simulink model "TBRe18_ECU_V6"  (R2015b)
settings: Solver=FixedStepDiscrete  SolverMode=SingleTasking  StartTime=0.0  StopTime=inf  FixedStep=0.0001  RelTol=1e-3
PostLoadFcn:
  | model_init();
libraries: simulink x20, simulink_extras x1
(part 3 of 4)

== system TBRe18_ECU_V6/Low_Priority_CAN_TX/ECU_Data ==
  In1 : Inport
  Bus Selector : BusSelector  OutputSignals=Input_Data_Bus.BMS_Data.Pre_Charge_Hold,Vehicle_Operation_Data.Throttle_Bool,Vehicle_Operation_Data.MCU_NMT_Mode,Vehicle_Operation_Data.PWM,Vehicle_Operation_Data.Buzzer,Vehicle_Operation_Data.Operation_Mode,Vehicle_Operation_Data.Brake_Bool
  Bus Selector1 : BusSelector  OutputSignals=Input_Data_Bus.ECU_IO_Data.Pedal_Box_Data.Brake_Voltage,Input_Data_Bus.ECU_IO_Data.Pedal_Box_Data.Throttle2_Voltage,Input_Data_Bus.ECU_IO_Data.Pedal_Box_Data.Throttle1_Voltage,Input_Data_Bus.ECU_IO_Data.Pedal_Box_Data.Throttle_%,Input_Data_Bus.ECU_IO_Data.Pedal_Box_Data.APPS_Implausibility,Input_Data_Bus.ECU_IO_Data.Pedal_Box_Data.APPS_BP_Implausibility,Input_Data_Bus.ECU_IO_Data.Pedal_Box_Data.Brake_%,Input_Data_Bus.ECU_IO_Data.Pedal_Box_Data.Throttle2_%,Input_Data_Bus.ECU_IO_Data.Pedal_Box_Data.Throttle1_%,Input_Data_Bus.ECU_IO_Data.Pedal_Box_Data.Pedal_Sensor_Fail,Input_Data_Bus.ECU_IO_Data.LV_Battery_Data.LV_Battery_Warning,Input_Data_Bus.ECU_IO_Data.LV_Battery_Data.LV_Battery_SOC,Input_Data_Bus.ECU_IO_Data.LV_Battery_Data.LV_Battery_Voltage,Input_Data_Bus.Raw_Input_Data.Hardwired_Inputs.Console_Data.Push_to_Start,Input_Data_Bus.Raw_Input_Data.Hardwired_Inputs.Console_Data.Reset
  Bus Selector2 : BusSelector  OutputSignals=Input_Data_Bus.BMS_Data.IMD_Fault,Input_Data_Bus.MCU_Data.MCU_Error,Input_Data_Bus.Raw_Input_Data.LP_CAN_RX.Shutdown_Data.BMS_Fault,Input_Data_Bus.ECU_IO_Data.Pedal_Box_Data.APPS_Implausibility,Input_Data_Bus.ECU_IO_Data.Pedal_Box_Data.APPS_BP_Implausibility,Input_Data_Bus.Shutdown_Data.Shutdown_Error,Input_Data_Bus.ECU_IO_Data.LV_Battery_Data.LV_Battery_Warning
  CanTx : S-Function  FunctionName=NsiCan_Tx  Parameters=data_can,channel,msg_name,ident,ident_type,dlc,signals  SFunctionDeploymentMode=off  EnableBusSupport=off  mask(MUXlink Can Tx){data_can=1;HIGH_SPEED;500Kbps;120 Ohm;C:\Users\William\Documents\ECU\DBC\TBRe18_DBC_V1.dbc;0;1;HIGH_SPEED;500Kbps;120 Ohm;C:\Users\William\Documents\ECU\DBC\TBRe18_DBC_V1.dbc;0;0;HIGH_SPEED;500Kbps;120 Ohm;C:\Users\l\Desktop\FYP\ECU\DBC\TBRe_DBC_V2.dbc;0;0;HIGH_SPEED;500Kbps;120 Ohm;D:\TOOLS\MUXLINK\R2011b\MUXlink\misc\j1939_adapt.dbc;0;0;HIGH_SPEED;1000Kbps;No;D:\TOOLS\MUXLINK\R2011b\MUXlink\misc\BASE_CAN_MUXLAB4.dbc;0, channel=2, msg_name=ECU_Pedal_Box_Data, ident=0x702, ident_type=STD, dlc=5, signals=Throttle_Percentage;1;32;8;APPS_Implausibility;1;4;1;APPS_BP_Implausibility;1;3;1;Brake_Percentage;1;24;8;Throttle2_Percentage;1;16;8;Throttle1_Percent;1;8;8;Pedal_Sensor_Fail;1;0;3}
      mask prompts: data_can "data can"; msg_name "msg name"
      mask help: Transmit a frame on a CAN Channel.
      mask init:
      | NsiCan_Tx_InitializationFcn();
      settings: OpenFcn=NsiCan_Tx_OpenFcn();
      mask Help:
      | eval('block=get_param(gcb, ''RTWdata'');')
      | web([docroot '\toolbox\MUXlink\html\blocks/' block.MUXlink_BlockType '.html'])
      mask Callback data_can: NsiCan_Tx_ApplyFcn(1);
      mask Callback channel: NsiCan_Tx_ApplyFcn(2);
      mask Callback msg_name: NsiCan_Tx_ApplyFcn(3);
      mask Callback ident: NsiCan_Tx_ApplyFcn(4);
      mask Callback ident_type: NsiCan_Tx_ApplyFcn(5);
      mask Callback dlc: NsiCan_Tx_ApplyFcn(6);
      mask Callback signals: NsiCan_Tx_ApplyFcn(7);
      mask Display: image(imread('nsi.bmp'));text(0.5, 0.1, 'TX_ECU_Pedal_Box_Data_CAN2', 'horizontalAlignment', 'center', 'verticalAlignment', 'base');plot([0.05 0.05 0.05 0.05 0.05 0.05 0.05 0.05 0.05 0.05]); port_label('input',1, 'Throttle_Percentage'); port_label('input',2, 'APPS_Implausibility'); port_label('input',3, 'APPS_BP_Implausibility'); port_label('input',4, 'Brake_Percentage'); port_label('input',5, 'Throttle2_Percentage'); port_label('input',6, 'Throttle1_Percent'); port_label('input',7, 'Pedal_Sensor_Fail');
  CanTx1 : S-Function  FunctionName=NsiCan_Tx  Parameters=data_can,channel,msg_name,ident,ident_type,dlc,signals  SFunctionDeploymentMode=off  EnableBusSupport=off  mask(MUXlink Can Tx){data_can=1;HIGH_SPEED;500Kbps;120 Ohm;C:\Users\William\Documents\ECU\DBC\TBRe18_DBC_V1.dbc;0;1;HIGH_SPEED;500Kbps;120 Ohm;C:\Users\William\Documents\ECU\DBC\TBRe18_DBC_V1.dbc;0;0;HIGH_SPEED;500Kbps;120 Ohm;C:\Users\l\Desktop\FYP\ECU\DBC\TBRe_DBC_V2.dbc;0;0;HIGH_SPEED;500Kbps;120 Ohm;D:\TOOLS\MUXLINK\R2011b\MUXlink\misc\j1939_adapt.dbc;0;0;HIGH_SPEED;1000Kbps;No;D:\TOOLS\MUXLINK\R2011b\MUXlink\misc\BASE_CAN_MUXLAB4.dbc;0, channel=2, msg_name=ECU_Pedal_Voltages, ident=0x703, ident_type=STD, dlc=8, signals=Brake_Voltage;1;32;16;Throttle2_Voltage;1;48;16;Throttle1_Voltage;1;0;16}
      mask prompts: data_can "data can"; msg_name "msg name"
      mask help: Transmit a frame on a CAN Channel.
      mask init:
      | NsiCan_Tx_InitializationFcn();
      settings: OpenFcn=NsiCan_Tx_OpenFcn();
      mask Help:
      | eval('block=get_param(gcb, ''RTWdata'');')
      | web([docroot '\toolbox\MUXlink\html\blocks/' block.MUXlink_BlockType '.html'])
      mask Callback data_can: NsiCan_Tx_ApplyFcn(1);
      mask Callback channel: NsiCan_Tx_ApplyFcn(2);
      mask Callback msg_name: NsiCan_Tx_ApplyFcn(3);
      mask Callback ident: NsiCan_Tx_ApplyFcn(4);
      mask Callback ident_type: NsiCan_Tx_ApplyFcn(5);
      mask Callback dlc: NsiCan_Tx_ApplyFcn(6);
      mask Callback signals: NsiCan_Tx_ApplyFcn(7);
      mask Display: image(imread('nsi.bmp'));text(0.5, 0.1, 'TX_ECU_Pedal_Voltages_CAN2', 'horizontalAlignment', 'center', 'verticalAlignment', 'base');plot([0.05 0.05 0.05 0.05 0.05 0.05 0.05 0.05 0.05 0.05]); port_label('input',1, 'Brake_Voltage'); port_label('input',2, 'Throttle2_Voltage'); port_label('input',3, 'Throttle1_Voltage');
  CanTx2 : S-Function  FunctionName=NsiCan_Tx  Parameters=data_can,channel,msg_name,ident,ident_type,dlc,signals  SFunctionDeploymentMode=off  EnableBusSupport=off  mask(MUXlink Can Tx){data_can=1;HIGH_SPEED;500Kbps;120 Ohm;C:\Users\William\Documents\ECU\DBC\TBRe18_DBC_V1.dbc;0;1;HIGH_SPEED;500Kbps;120 Ohm;C:\Users\William\Documents\ECU\DBC\TBRe18_DBC_V1.dbc;0;0;HIGH_SPEED;500Kbps;120 Ohm;C:\Users\l\Desktop\FYP\ECU\DBC\TBRe_DBC_V2.dbc;0;0;HIGH_SPEED;500Kbps;120 Ohm;D:\TOOLS\MUXLINK\R2011b\MUXlink\misc\j1939_adapt.dbc;0;0;HIGH_SPEED;1000Kbps;No;D:\TOOLS\MUXLINK\R2011b\MUXlink\misc\BASE_CAN_MUXLAB4.dbc;0, channel=2, msg_name=ECU_HW_IO, ident=0x282, ident_type=STD, dlc=4, signals=LV_Battery_Warning;1;10;1;LV_Battery_SOC;1;0;8;LV_Battery_Voltage;1;16;16;Console_Push_to_Start;1;9;1;Console_Reset;1;8;1}
      mask prompts: data_can "data can"; msg_name "msg name"
      mask help: Transmit a frame on a CAN Channel.
      mask init:
      | NsiCan_Tx_InitializationFcn();
      settings: OpenFcn=NsiCan_Tx_OpenFcn();
      mask Help:
      | eval('block=get_param(gcb, ''RTWdata'');')
      | web([docroot '\toolbox\MUXlink\html\blocks/' block.MUXlink_BlockType '.html'])
      mask Callback data_can: NsiCan_Tx_ApplyFcn(1);
      mask Callback channel: NsiCan_Tx_ApplyFcn(2);
      mask Callback msg_name: NsiCan_Tx_ApplyFcn(3);
      mask Callback ident: NsiCan_Tx_ApplyFcn(4);
      mask Callback ident_type: NsiCan_Tx_ApplyFcn(5);
      mask Callback dlc: NsiCan_Tx_ApplyFcn(6);
      mask Callback signals: NsiCan_Tx_ApplyFcn(7);
      mask Display: image(imread('nsi.bmp'));text(0.5, 0.1, 'TX_ECU_HW_IO_CAN2', 'horizontalAlignment', 'center', 'verticalAlignment', 'base');plot([0.05 0.05 0.05 0.05 0.05 0.05 0.05 0.05 0.05 0.05]); port_label('input',1, 'LV_Battery_Warning'); port_label('input',2, 'LV_Battery_SOC'); port_label('input',3, 'LV_Battery_Voltage'); port_label('input',4, 'Console_Push_to_Start'); port_label('input',5, 'Console_Reset');
  CanTx3 : S-Function  FunctionName=NsiCan_Tx  Parameters=data_can,channel,msg_name,ident,ident_type,dlc,signals  SFunctionDeploymentMode=off  EnableBusSupport=off  mask(MUXlink Can Tx){data_can=1;HIGH_SPEED;500Kbps;120 Ohm;C:\Users\William\Documents\ECU\DBC\TBRe18_DBC_V1.dbc;0;1;HIGH_SPEED;500Kbps;120 Ohm;C:\Users\William\Documents\ECU\DBC\TBRe18_DBC_V1.dbc;0;0;HIGH_SPEED;500Kbps;120 Ohm;C:\Users\l\Desktop\FYP\ECU\DBC\TBRe_DBC_V2.dbc;0;0;HIGH_SPEED;500Kbps;120 Ohm;D:\TOOLS\MUXLINK\R2011b\MUXlink\misc\j1939_adapt.dbc;0;0;HIGH_SPEED;1000Kbps;No;D:\TOOLS\MUXLINK\R2011b\MUXlink\misc\BASE_CAN_MUXLAB4.dbc;0, channel=2, msg_name=ECU_Vehicle_Functionality, ident=0x704, ident_type=STD, dlc=4, signals=Pre_Charge;1;24;8;Throttle_Bool;1;2;1;MCU_NMT_Mode;1;16;8;PWM;1;3;1;Buzzer;1;1;1;Vehicle_Operation;1;8;8;Brake_Bool;1;0;1}
      mask prompts: data_can "data can"; msg_name "msg name"
      mask help: Transmit a frame on a CAN Channel.
      mask init:
      | NsiCan_Tx_InitializationFcn();
      settings: OpenFcn=NsiCan_Tx_OpenFcn();
      mask Help:
      | eval('block=get_param(gcb, ''RTWdata'');')
      | web([docroot '\toolbox\MUXlink\html\blocks/' block.MUXlink_BlockType '.html'])
      mask Callback data_can: NsiCan_Tx_ApplyFcn(1);
      mask Callback channel: NsiCan_Tx_ApplyFcn(2);
      mask Callback msg_name: NsiCan_Tx_ApplyFcn(3);
      mask Callback ident: NsiCan_Tx_ApplyFcn(4);
      mask Callback ident_type: NsiCan_Tx_ApplyFcn(5);
      mask Callback dlc: NsiCan_Tx_ApplyFcn(6);
      mask Callback signals: NsiCan_Tx_ApplyFcn(7);
      mask Display: image(imread('nsi.bmp'));text(0.5, 0.1, 'TX_ECU_Vehicle_Functionality_CAN2', 'horizontalAlignment', 'center', 'verticalAlignment', 'base');plot([0.05 0.05 0.05 0.05 0.05 0.05 0.05 0.05 0.05 0.05]); port_label('input',1, 'Pre_Charge'); port_label('input',2, 'Throttle_Bool'); port_label('input',3, 'MCU_NMT_Mode'); port_label('input',4, 'PWM'); port_label('input',5, 'Buzzer'); port_label('input',6, 'Vehicle_Operation'); port_label('input',7, 'Brake_Bool');
  CanTx4 : S-Function  FunctionName=NsiCan_Tx  Parameters=data_can,channel,msg_name,ident,ident_type,dlc,signals  SFunctionDeploymentMode=off  EnableBusSupport=off  mask(MUXlink Can Tx){data_can=1;HIGH_SPEED;500Kbps;120 Ohm;C:\Users\William\Documents\ECU\DBC\TBRe18_DBC_V1.dbc;0;1;HIGH_SPEED;500Kbps;120 Ohm;C:\Users\William\Documents\ECU\DBC\TBRe18_DBC_V1.dbc;0;0;HIGH_SPEED;500Kbps;120 Ohm;C:\Users\l\Desktop\FYP\ECU\DBC\TBRe_DBC_V2.dbc;0;0;HIGH_SPEED;500Kbps;120 Ohm;D:\TOOLS\MUXLINK\R2011b\MUXlink\misc\j1939_adapt.dbc;0;0;HIGH_SPEED;1000Kbps;No;D:\TOOLS\MUXLINK\R2011b\MUXlink\misc\BASE_CAN_MUXLAB4.dbc;0, channel=2, msg_name=ECU_Diagnostics, ident=0x700, ident_type=STD, dlc=4, signals=IMD_Fault;1;13;1;MCU_TPDO1_ErrorCode;1;16;16;BMS_Fault;1;5;1;APPS_Implausibility;1;4;1;APPS_BP_Implausibility;1;3;1;Shutdown_Error;1;2;1;LV_Battery_Warning;1;1;1}
      mask prompts: data_can "data can"; msg_name "msg name"
      mask help: Transmit a frame on a CAN Channel.
      mask init:
      | NsiCan_Tx_InitializationFcn();
      settings: OpenFcn=NsiCan_Tx_OpenFcn();
      mask Help:
      | eval('block=get_param(gcb, ''RTWdata'');')
      | web([docroot '\toolbox\MUXlink\html\blocks/' block.MUXlink_BlockType '.html'])
      mask Callback data_can: NsiCan_Tx_ApplyFcn(1);
      mask Callback channel: NsiCan_Tx_ApplyFcn(2);
      mask Callback msg_name: NsiCan_Tx_ApplyFcn(3);
      mask Callback ident: NsiCan_Tx_ApplyFcn(4);
      mask Callback ident_type: NsiCan_Tx_ApplyFcn(5);
      mask Callback dlc: NsiCan_Tx_ApplyFcn(6);
      mask Callback signals: NsiCan_Tx_ApplyFcn(7);
      mask Display: image(imread('nsi.bmp'));text(0.5, 0.1, 'TX_ECU_Diagnostics_CAN2', 'horizontalAlignment', 'center', 'verticalAlignment', 'base');plot([0.05 0.05 0.05 0.05 0.05 0.05 0.05 0.05 0.05 0.05]); port_label('input',1, 'IMD_Fault'); port_label('input',2, 'MCU_TPDO1_ErrorCode'); port_label('input',3, 'BMS_Fault'); port_label('input',4, 'APPS_Implausibility'); port_label('input',5, 'APPS_BP_Implausibility'); port_label('input',6, 'Shutdown_Error'); port_label('input',7, 'LV_Battery_Warning');
  Data Type Conversion : DataTypeConversion  OutDataTypeStr=uint8
  wires:
  Bus Selector1/2 -> CanTx1/2  "<Throttle2_Voltage>"
  Bus Selector1/3 -> CanTx1/3  "<Throttle1_Voltage>"
  Bus Selector1/4 -> CanTx/1  "<Throttle_%>"
  Bus Selector1/5 -> CanTx/2  "<APPS_Implausibility>"
  Bus Selector1/6 -> CanTx/3  "<APPS_BP_Implausibility>"
  Bus Selector1/11 -> CanTx2/1  "<LV_Battery_Warning>"
  Bus Selector1/12 -> CanTx2/2  "<LV_Battery_SOC>"
  Bus Selector1/13 -> CanTx2/3  "<LV_Battery_Voltage>"
  Bus Selector1/14 -> CanTx2/4  "<Push_to_Start>"
  Bus Selector1/15 -> CanTx2/5  "<Reset>"
  In1/1 -> Bus Selector2/1, Bus Selector/1, Bus Selector1/1
  Bus Selector1/1 -> CanTx1/1  "<Brake_Voltage>"
  Bus Selector1/7 -> CanTx/4  "<Brake_%>"
  Bus Selector1/10 -> CanTx/7  "<Pedal_Sensor_Fail>"
  Bus Selector1/8 -> CanTx/5  "<Throttle2_%>"
  Bus Selector1/9 -> CanTx/6  "<Throttle1_%>"
  Bus Selector2/1 -> CanTx4/1  "<IMD_Fault>"
  Bus Selector2/2 -> CanTx4/2  "<MCU_Error>"
  Bus Selector2/3 -> CanTx4/3  "<BMS_Fault>"
  Bus Selector2/4 -> CanTx4/4  "<APPS_Implausibility>"
  Bus Selector2/5 -> CanTx4/5  "<APPS_BP_Implausibility>"
  Bus Selector2/6 -> CanTx4/6  "<Shutdown_Error>"
  Bus Selector2/7 -> CanTx4/7  "<LV_Battery_Warning>"
  Bus Selector/2 -> CanTx3/2  "<Throttle_Bool>"
  Bus Selector/3 -> CanTx3/3  "<MCU_NMT_Mode>"
  Bus Selector/4 -> CanTx3/4  "<PWM>"
  Bus Selector/5 -> CanTx3/5  "<Buzzer>"
  Bus Selector/6 -> CanTx3/6  "<Operation_Mode>"
  Bus Selector/7 -> CanTx3/7  "<Brake_Bool>"
  Bus Selector/1 -> Data Type Conversion/1  "<Pre_Charge_Hold>"
  Data Type Conversion/1 -> CanTx3/1

== system TBRe18_ECU_V6/Low_Priority_CAN_TX/Init ==

== system TBRe18_ECU_V6/Low_Priority_CAN_TX/MCU_Data ==
  In1 : Inport
  Bus Selector : BusSelector  OutputSignals=Input_Data_Bus.MCU_Data.DC_Link_Current,Input_Data_Bus.MCU_Data.DC_Link_Voltage,Input_Data_Bus.MCU_Data.Motor_Temp,Input_Data_Bus.MCU_Data.MCU_Temp
  CanRx : S-Function  FunctionName=NsiCan_Rx  Parameters=data_can,channel,msg_name,ident,ident_type,dlc,signals,is_trigger  SFunctionDeploymentMode=off  EnableBusSupport=off  mask(MUXlink Can Rx){data_can=1;HIGH_SPEED;500Kbps;120 Ohm;C:\Users\William\Documents\ECU\DBC\TBRe18_DBC_V1.dbc;0;;1;HIGH_SPEED;500Kbps;120 Ohm;C:\Users\William\Documents\ECU\DBC\TBRe18_DBC_V1.dbc;0;;0;HIGH_SPEED;500Kbps;120 Ohm;C:\Users\l\Desktop\FYP\ECU\DBC\TBRe_DBC_V2.dbc;0;;0;HIGH_SPEED;500Kbps;120 Ohm;D:\TOOLS\MUXLINK\R2011b\MUXlink\misc\j1939_adapt.dbc;0;;0;HIGH_SPEED;1000Kbps;No;D:\TOOLS\MUXLINK\R2011b\MUXlink\misc\BASE_CAN_MUXLAB4.dbc;0;, channel=1, msg_name=MCU_TPDO4, ident=0x481, ident_type=STD, dlc=8, signals=MCU_DC_Power;1;0;-32;MCU_Velocity_Actual_Value;1;32;-32, is_trigger=0}
      mask prompts: data_can "data can"; msg_name "msg name"
      mask help: Receive a frame from a CAN channel.
      mask init:
      | NsiCan_Rx_InitializationFcn();
      settings: OpenFcn=NsiCan_Rx_OpenFcn();
      mask Help:
      | eval('block=get_param(gcb, ''RTWdata'');')
      | web([docroot '\toolbox\MUXlink\html\blocks/' block.MUXlink_BlockType '.html'])
      mask Callback data_can: NsiCan_Rx_ApplyFcn(1);
      mask Callback channel: NsiCan_Rx_ApplyFcn(2);
      mask Callback msg_name: NsiCan_Rx_ApplyFcn(3);
      mask Callback ident: NsiCan_Rx_ApplyFcn(4);
      mask Callback ident_type: NsiCan_Rx_ApplyFcn(5);
      mask Callback dlc: NsiCan_Rx_ApplyFcn(6);
      mask Callback signals: NsiCan_Rx_ApplyFcn(7);
      mask Callback is_trigger: NsiCan_Rx_ApplyFcn(8);
      mask Display: image(imread('nsi.bmp'));text(0.5, 0.3, 'RX_MCU_TPDO4_CAN1', 'horizontalAlignment', 'center', 'verticalAlignment', 'base');plot([0.05 0.05 0.05 0.05 0.05 0.05 0.05 0.05 0.05 0.05]); port_label('output',1, 'MCU_DC_Power'); port_label('output',2, 'MCU_Velocity_Actual_Value'); port_label('output',3, 'Status');
  CanRx1 : S-Function  FunctionName=NsiCan_Rx  Parameters=data_can,channel,msg_name,ident,ident_type,dlc,signals,is_trigger  SFunctionDeploymentMode=off  EnableBusSupport=off  mask(MUXlink Can Rx){data_can=1;HIGH_SPEED;500Kbps;120 Ohm;C:\Users\William\Documents\ECU\DBC\TBRe18_DBC_V1.dbc;0;;1;HIGH_SPEED;500Kbps;120 Ohm;C:\Users\William\Documents\ECU\DBC\TBRe18_DBC_V1.dbc;0;;0;HIGH_SPEED;500Kbps;120 Ohm;C:\Users\l\Desktop\FYP\ECU\DBC\TBRe_DBC_V2.dbc;0;;0;HIGH_SPEED;500Kbps;120 Ohm;D:\TOOLS\MUXLINK\R2011b\MUXlink\misc\j1939_adapt.dbc;0;;0;HIGH_SPEED;1000Kbps;No;D:\TOOLS\MUXLINK\R2011b\MUXlink\misc\BASE_CAN_MUXLAB4.dbc;0;, channel=1, msg_name=MCU_TPDO3, ident=0x381, ident_type=STD, dlc=8, signals=MCU_Error_Code;1;0;-16;MCU_Status_Word;1;16;16;MCU_PhaseB_Current;1;48;-16;MCU_PhaseA_Current;1;32;-16, is_trigger=0}
      mask prompts: data_can "data can"; msg_name "msg name"
      mask help: Receive a frame from a CAN channel.
      mask init:
      | NsiCan_Rx_InitializationFcn();
      settings: OpenFcn=NsiCan_Rx_OpenFcn();
      mask Help:
      | eval('block=get_param(gcb, ''RTWdata'');')
      | web([docroot '\toolbox\MUXlink\html\blocks/' block.MUXlink_BlockType '.html'])
      mask Callback data_can: NsiCan_Rx_ApplyFcn(1);
      mask Callback channel: NsiCan_Rx_ApplyFcn(2);
      mask Callback msg_name: NsiCan_Rx_ApplyFcn(3);
      mask Callback ident: NsiCan_Rx_ApplyFcn(4);
      mask Callback ident_type: NsiCan_Rx_ApplyFcn(5);
      mask Callback dlc: NsiCan_Rx_ApplyFcn(6);
      mask Callback signals: NsiCan_Rx_ApplyFcn(7);
      mask Callback is_trigger: NsiCan_Rx_ApplyFcn(8);
      mask Display: image(imread('nsi.bmp'));text(0.5, 0.3, 'RX_MCU_TPDO3_CAN1', 'horizontalAlignment', 'center', 'verticalAlignment', 'base');plot([0.05 0.05 0.05 0.05 0.05 0.05 0.05 0.05 0.05 0.05]); port_label('output',1, 'MCU_Error_Code'); port_label('output',2, 'MCU_Status_Word'); port_label('output',3, 'MCU_PhaseB_Current'); port_label('output',4, 'MCU_PhaseA_Current'); port_label('output',5, 'Status');
  CanTx : S-Function  FunctionName=NsiCan_Tx  Parameters=data_can,channel,msg_name,ident,ident_type,dlc,signals  SFunctionDeploymentMode=off  EnableBusSupport=off  mask(MUXlink Can Tx){data_can=1;HIGH_SPEED;500Kbps;120 Ohm;C:\Users\William\Documents\ECU\DBC\TBRe18_DBC_V1.dbc;0;1;HIGH_SPEED;500Kbps;120 Ohm;C:\Users\William\Documents\ECU\DBC\TBRe18_DBC_V1.dbc;0;0;HIGH_SPEED;500Kbps;120 Ohm;C:\Users\l\Desktop\FYP\ECU\DBC\TBRe_DBC_V2.dbc;0;0;HIGH_SPEED;500Kbps;120 Ohm;D:\TOOLS\MUXLINK\R2011b\MUXlink\misc\j1939_adapt.dbc;0;0;HIGH_SPEED;1000Kbps;No;D:\TOOLS\MUXLINK\R2011b\MUXlink\misc\BASE_CAN_MUXLAB4.dbc;0, channel=2, msg_name=MCU_TPDO4, ident=0x481, ident_type=STD, dlc=8, signals=MCU_DC_Power;1;0;-32;MCU_Velocity_Actual_Value;1;32;-32}
      mask prompts: data_can "data can"; msg_name "msg name"
      mask help: Transmit a frame on a CAN Channel.
      mask init:
      | NsiCan_Tx_InitializationFcn();
      settings: OpenFcn=NsiCan_Tx_OpenFcn();
      mask Help:
      | eval('block=get_param(gcb, ''RTWdata'');')
      | web([docroot '\toolbox\MUXlink\html\blocks/' block.MUXlink_BlockType '.html'])
      mask Callback data_can: NsiCan_Tx_ApplyFcn(1);
      mask Callback channel: NsiCan_Tx_ApplyFcn(2);
      mask Callback msg_name: NsiCan_Tx_ApplyFcn(3);
      mask Callback ident: NsiCan_Tx_ApplyFcn(4);
      mask Callback ident_type: NsiCan_Tx_ApplyFcn(5);
      mask Callback dlc: NsiCan_Tx_ApplyFcn(6);
      mask Callback signals: NsiCan_Tx_ApplyFcn(7);
      mask Display: image(imread('nsi.bmp'));text(0.5, 0.3, 'TX_MCU_TPDO4_CAN2', 'horizontalAlignment', 'center', 'verticalAlignment', 'base');plot([0.05 0.05 0.05 0.05 0.05 0.05 0.05 0.05 0.05 0.05]); port_label('input',1, 'MCU_DC_Power'); port_label('input',2, 'MCU_Velocity_Actual_Value');
  CanTx1 : S-Function  FunctionName=NsiCan_Tx  Parameters=data_can,channel,msg_name,ident,ident_type,dlc,signals  SFunctionDeploymentMode=off  EnableBusSupport=off  mask(MUXlink Can Tx){data_can=1;HIGH_SPEED;500Kbps;120 Ohm;C:\Users\William\Documents\ECU\DBC\TBRe18_DBC_V1.dbc;0;1;HIGH_SPEED;500Kbps;120 Ohm;C:\Users\William\Documents\ECU\DBC\TBRe18_DBC_V1.dbc;0;0;HIGH_SPEED;500Kbps;120 Ohm;C:\Users\l\Desktop\FYP\ECU\DBC\TBRe_DBC_V2.dbc;0;0;HIGH_SPEED;500Kbps;120 Ohm;D:\TOOLS\MUXLINK\R2011b\MUXlink\misc\j1939_adapt.dbc;0;0;HIGH_SPEED;1000Kbps;No;D:\TOOLS\MUXLINK\R2011b\MUXlink\misc\BASE_CAN_MUXLAB4.dbc;0, channel=2, msg_name=MCU_TPDO3, ident=0x381, ident_type=STD, dlc=8, signals=MCU_Error_Code;1;0;-16;MCU_Status_Word;1;16;16;MCU_PhaseB_Current;1;48;-16;MCU_PhaseA_Current;1;32;-16}
      mask prompts: data_can "data can"; msg_name "msg name"
      mask help: Transmit a frame on a CAN Channel.
      mask init:
      | NsiCan_Tx_InitializationFcn();
      settings: OpenFcn=NsiCan_Tx_OpenFcn();
      mask Help:
      | eval('block=get_param(gcb, ''RTWdata'');')
      | web([docroot '\toolbox\MUXlink\html\blocks/' block.MUXlink_BlockType '.html'])
      mask Callback data_can: NsiCan_Tx_ApplyFcn(1);
      mask Callback channel: NsiCan_Tx_ApplyFcn(2);
      mask Callback msg_name: NsiCan_Tx_ApplyFcn(3);
      mask Callback ident: NsiCan_Tx_ApplyFcn(4);
      mask Callback ident_type: NsiCan_Tx_ApplyFcn(5);
      mask Callback dlc: NsiCan_Tx_ApplyFcn(6);
      mask Callback signals: NsiCan_Tx_ApplyFcn(7);
      mask Display: image(imread('nsi.bmp'));text(0.5, 0.3, 'TX_MCU_TPDO3_CAN2', 'horizontalAlignment', 'center', 'verticalAlignment', 'base');plot([0.05 0.05 0.05 0.05 0.05 0.05 0.05 0.05 0.05 0.05]); port_label('input',1, 'MCU_Error_Code'); port_label('input',2, 'MCU_Status_Word'); port_label('input',3, 'MCU_PhaseB_Current'); port_label('input',4, 'MCU_PhaseA_Current');
  CanTx2 : S-Function  FunctionName=NsiCan_Tx  Parameters=data_can,channel,msg_name,ident,ident_type,dlc,signals  SFunctionDeploymentMode=off  EnableBusSupport=off  mask(MUXlink Can Tx){data_can=1;HIGH_SPEED;500Kbps;120 Ohm;C:\Users\William\Documents\ECU\DBC\TBRe18_DBC_V1.dbc;0;1;HIGH_SPEED;500Kbps;120 Ohm;C:\Users\William\Documents\ECU\DBC\TBRe18_DBC_V1.dbc;0;0;HIGH_SPEED;500Kbps;120 Ohm;C:\Users\l\Desktop\FYP\ECU\DBC\TBRe_DBC_V2.dbc;0;0;HIGH_SPEED;500Kbps;120 Ohm;D:\TOOLS\MUXLINK\R2011b\MUXlink\misc\j1939_adapt.dbc;0;0;HIGH_SPEED;1000Kbps;No;D:\TOOLS\MUXLINK\R2011b\MUXlink\misc\BASE_CAN_MUXLAB4.dbc;0, channel=2, msg_name=MCU_TPDO2, ident=0x281, ident_type=STD, dlc=8, signals=MCU_DC_Link_Current;1;32;-32;MCU_DC_Link_Voltage;1;16;-16;Motor_Temp;1;8;8;MCU_Temp;1;0;8}
      mask prompts: data_can "data can"; msg_name "msg name"
      mask help: Transmit a frame on a CAN Channel.
      mask init:
      | NsiCan_Tx_InitializationFcn();
      settings: OpenFcn=NsiCan_Tx_OpenFcn();
      mask Help:
      | eval('block=get_param(gcb, ''RTWdata'');')
      | web([docroot '\toolbox\MUXlink\html\blocks/' block.MUXlink_BlockType '.html'])
      mask Callback data_can: NsiCan_Tx_ApplyFcn(1);
      mask Callback channel: NsiCan_Tx_ApplyFcn(2);
      mask Callback msg_name: NsiCan_Tx_ApplyFcn(3);
      mask Callback ident: NsiCan_Tx_ApplyFcn(4);
      mask Callback ident_type: NsiCan_Tx_ApplyFcn(5);
      mask Callback dlc: NsiCan_Tx_ApplyFcn(6);
      mask Callback signals: NsiCan_Tx_ApplyFcn(7);
      mask Display: image(imread('nsi.bmp'));text(0.5, 0.3, 'TX_MCU_TPDO2_CAN2', 'horizontalAlignment', 'center', 'verticalAlignment', 'base');plot([0.05 0.05 0.05 0.05 0.05 0.05 0.05 0.05 0.05 0.05]); port_label('input',1, 'MCU_DC_Link_Current'); port_label('input',2, 'MCU_DC_Link_Voltage'); port_label('input',3, 'Motor_Temp'); port_label('input',4, 'MCU_Temp');
  wires:
  CanRx/1 -> CanTx/1
  CanRx/2 -> CanTx/2
  CanRx1/1 -> CanTx1/1
  CanRx1/2 -> CanTx1/2
  CanRx1/3 -> CanTx1/3
  CanRx1/4 -> CanTx1/4
  Bus Selector/1 -> CanTx2/1  "<DC_Link_Current>"
  Bus Selector/2 -> CanTx2/2  "<DC_Link_Voltage>"
  Bus Selector/3 -> CanTx2/3  "<Motor_Temp>"
  Bus Selector/4 -> CanTx2/4  "<MCU_Temp>"
  In1/1 -> Bus Selector/1

== system TBRe18_ECU_V6/Low_Priority_CAN_TX/Shutdown_System_Data ==
  In1 : Inport

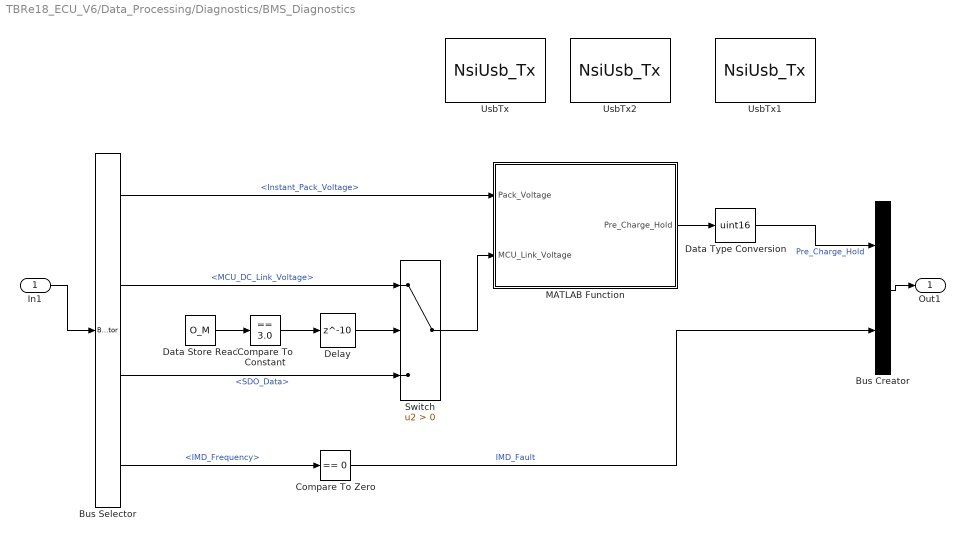
== system TBRe18_ECU_V6/Data_Processing/Diagnostics/BMS_Diagnostics ==
  In1 : Inport
  Bus Creator : BusCreator  Inputs=2
  Bus Selector : BusSelector  OutputSignals=LP_CAN_RX.BMS_Data.Instant_Pack_Voltage,HP_CAN_RX.MCU_DC_Link_Voltage,HP_CAN_RX.SDO_Data,Hardwired_Inputs.IMD_Frequency
  Compare To Constant : simulink/Logic and Bit Operations/Compare To Constant  relop===  const=3.0  OutDataTypeStr=boolean
  Compare To Zero : simulink/Logic and Bit Operations/Compare To Zero  relop===  OutDataTypeStr=boolean
  Data Store Read : DataStoreRead  DataStoreName=O_M
  Data Type Conversion : DataTypeConversion  OutDataTypeStr=uint16
  Delay : Delay  DelayLength=10  InitialCondition=0
  MATLAB Function : MATLAB Function  TreatAsAtomicUnit=on
  Switch : Switch  Criteria=u2 > Threshold
  UsbTx : S-Function  FunctionName=NsiUsb_Tx  Parameters=signame,resolution,offset,unite  SFunctionDeploymentMode=off  EnableBusSupport=off  mask(MUXlink Usb Tx){signame=PACK, resolution=1, offset=0, unite=V}
      mask prompts: signame "Signal name ?"; resolution "Resolution ?"; offset "Offset ?"; unite "Unit ?"
      mask help: Transmit a frame on the USB Channel.
      mask init:
      | NsiUsb_Tx_InitializationFcn();
      settings: OpenFcn=NsiUsb_Tx_OpenFcn();
      mask Help:
      | eval('block=get_param(gcb, ''RTWdata'');')
      | web([docroot '\toolbox\MUXlink\html\blocks/' block.MUXlink_BlockType '.html'])
      mask Callback signame: NsiUsb_Tx_ApplyFcn(1);
      mask Callback resolution: NsiUsb_Tx_ApplyFcn(2);
      mask Callback offset: NsiUsb_Tx_ApplyFcn(3);
      mask Callback unite: NsiUsb_Tx_ApplyFcn(4);
      mask Display: image(imread('nsi.bmp'));text(0.5, 0.2, 'USB Tx', 'horizontalAlignment', 'center', 'verticalAlignment', 'base');plot([0.05 0.05 0.05 0.05 0.05 0.05 0.05 0.05 0.05 0.05]);port_label('input',1, 'PACK');
  UsbTx1 : S-Function  FunctionName=NsiUsb_Tx  Parameters=signame,resolution,offset,unite  SFunctionDeploymentMode=off  EnableBusSupport=off  mask(MUXlink Usb Tx){signame=MCU, resolution=1, offset=0, unite=V}
      mask prompts: signame "Signal name ?"; resolution "Resolution ?"; offset "Offset ?"; unite "Unit ?"
      mask help: Transmit a frame on the USB Channel.
      mask init:
      | NsiUsb_Tx_InitializationFcn();
      settings: OpenFcn=NsiUsb_Tx_OpenFcn();
      mask Help:
      | eval('block=get_param(gcb, ''RTWdata'');')
      | web([docroot '\toolbox\MUXlink\html\blocks/' block.MUXlink_BlockType '.html'])
      mask Callback signame: NsiUsb_Tx_ApplyFcn(1);
      mask Callback resolution: NsiUsb_Tx_ApplyFcn(2);
      mask Callback offset: NsiUsb_Tx_ApplyFcn(3);
      mask Callback unite: NsiUsb_Tx_ApplyFcn(4);
      mask Display: image(imread('nsi.bmp'));text(0.5, 0.2, 'USB Tx', 'horizontalAlignment', 'center', 'verticalAlignment', 'base');plot([0.05 0.05 0.05 0.05 0.05 0.05 0.05 0.05 0.05 0.05]);port_label('input',1, 'MCU');
  UsbTx2 : S-Function  FunctionName=NsiUsb_Tx  Parameters=signame,resolution,offset,unite  SFunctionDeploymentMode=off  EnableBusSupport=off  mask(MUXlink Usb Tx){signame=STATUS, resolution=1, offset=0, unite=V}
      mask prompts: signame "Signal name ?"; resolution "Resolution ?"; offset "Offset ?"; unite "Unit ?"
      mask help: Transmit a frame on the USB Channel.
      mask init:
      | NsiUsb_Tx_InitializationFcn();
      settings: OpenFcn=NsiUsb_Tx_OpenFcn();
      mask Help:
      | eval('block=get_param(gcb, ''RTWdata'');')
      | web([docroot '\toolbox\MUXlink\html\blocks/' block.MUXlink_BlockType '.html'])
      mask Callback signame: NsiUsb_Tx_ApplyFcn(1);
      mask Callback resolution: NsiUsb_Tx_ApplyFcn(2);
      mask Callback offset: NsiUsb_Tx_ApplyFcn(3);
      mask Callback unite: NsiUsb_Tx_ApplyFcn(4);
      mask Display: image(imread('nsi.bmp'));text(0.5, 0.2, 'USB Tx', 'horizontalAlignment', 'center', 'verticalAlignment', 'base');plot([0.05 0.05 0.05 0.05 0.05 0.05 0.05 0.05 0.05 0.05]);port_label('input',1, 'STATUS');
  Out1 : Outport
  wires:
  Bus Creator/1 -> Out1/1
  MATLAB Function/1(Pre_Charge_Hold) -> Data Type Conversion/1
  In1/1 -> Bus Selector/1
  Bus Selector/1 -> MATLAB Function/1(Pack_Voltage)  "<Instant_Pack_Voltage>"
  Data Type Conversion/1 -> Bus Creator/1  "Pre_Charge_Hold"
  Switch/1 -> MATLAB Function/2(MCU_Link_Voltage)
  Bus Selector/2 -> Switch/1  "<MCU_DC_Link_Voltage>"
  Bus Selector/3 -> Switch/3  "<SDO_Data>"
  Data Store Read/1 -> Compare To Constant/1
  Compare To Constant/1 -> Delay/1
  Delay/1 -> Switch/2
  Bus Selector/4 -> Compare To Zero/1  "<IMD_Frequency>"
  Compare To Zero/1 -> Bus Creator/2  "IMD_Fault"

== system TBRe18_ECU_V6/Data_Processing/Diagnostics/ECU_I//0s_Diagnostics ==
  In1 : Inport
  AIR : Subsystem
  Bus Creator : BusCreator  Inputs=4
  Bus Selector : BusSelector  OutputSignals=Hardwired_Inputs
  IMD : Subsystem
  LV_Battery : Subsystem
  Pedal_Box : Subsystem
  Out1 : Outport
  wires:
  In1/1 -> Bus Selector/1
  Bus Selector/1 -> LV_Battery/1(In1), Pedal_Box/1(In1), IMD/1(In1), AIR/1(In1)  "<Hardwired_Inputs>"
  Pedal_Box/1(Out1) -> Bus Creator/1  "Pedal_Box_Data"
  LV_Battery/1(Out1) -> Bus Creator/2  "LV_Battery_Data"
  IMD/1(Out1) -> Bus Creator/3  "IMD_Data"
  AIR/1(Out1) -> Bus Creator/4  "AIR_Data"
  Bus Creator/1 -> Out1/1

== system TBRe18_ECU_V6/Data_Processing/Diagnostics/MCU_Diagnostics ==
  In1 : Inport
  Bus Creator : BusCreator  Inputs=15
  Bus Selector : BusSelector  OutputSignals=HP_CAN_RX.Motor_Temp,HP_CAN_RX.MCU_Temp
  Bus Selector1 : BusSelector  OutputSignals=HP_CAN_RX.OD_Index,HP_CAN_RX.OD_Sub_Index,HP_CAN_RX.SDO_Data
  Configuration_Check : Subsystem  Commented=on
  Error_Check : simulink/Logic and Bit Operations/Compare To Zero  Commented=on  relop=~=  OutDataTypeStr=boolean
  MCU_Error : Logic  Commented=on  Operator=OR  AllPortsSameDT=off  OutDataTypeStr=boolean
  Power Monitoring : Subsystem  Commented=on
  Temp_Check : Subsystem
  Out1 : Outport
  wires:
  Bus Creator/1 -> Out1/1
  Error_Check/1 -> MCU_Error/1
  Temp_Check/1(MCU_Temperature) -> Bus Creator/7  "MCU_Temp"
  Temp_Check/2(Motor_Temperature) -> Bus Creator/8  "Motor_Temp"
  Temp_Check/3(MCU_Motor_Temp_Error) -> Bus Creator/9  "MCU_Motor_Temp_Error"
  Temp_Check/4(Coolant_Pump) -> Bus Creator/10  "Coolant_Pump"
  MCU_Error/1 -> Bus Creator/11  "MCU_Error"
  In1/1 -> Bus Selector1/1, Bus Selector/1
  Power Monitoring/1(MCU_Power) -> Bus Creator/12  "MCU_Power"
  Power Monitoring/2(DC_Link_Voltage) -> Bus Creator/13  "DC_Link_Voltage"
  Power Monitoring/3(DC_Link_Current) -> Bus Creator/14  "DC_Link_Current"
  Power Monitoring/4(Power_Limit_Breach) -> Bus Creator/15  "Power_Limit_Breach"
  Bus Selector1/1 -> Configuration_Check/1(OD_Index_In)  "<OD_Index>"
  Bus Selector1/2 -> Configuration_Check/2(OD_Sub_Index_In)  "<OD_Sub_Index>"
  Bus Selector1/3 -> Configuration_Check/3(SDO_Data_In)  "<SDO_Data>"
  Configuration_Check/1(SDO_Specifier) -> Bus Creator/1  "SDO_Specifier"
  Configuration_Check/2(OD_Index_Out) -> Bus Creator/2  "OD_Index_Out"
  Configuration_Check/3(OD_Sub_Index_Out) -> Bus Creator/3  "OD_Sub_Index"
  Configuration_Check/4(SDO_Data_Out) -> Bus Creator/4  "SDO_Data_Out"
  Configuration_Check/5(MCU_Config_Error) -> Bus Creator/5  "MCU_Config_Error"
  Bus Selector/1 -> Temp_Check/1(MCU_Temp)  "<Motor_Temp>"
  Configuration_Check/6(MCU_Config_Parameter_No) -> Bus Creator/6  "MCU_Config_Param_No"
  Bus Selector/2 -> Temp_Check/2(Motor_Temp)  "<MCU_Temp>"

== system TBRe18_ECU_V6/Data_Processing/Diagnostics/Shutdown_System_Diagnostics ==
  In1 : Inport
  Bus Creator : BusCreator  Inputs=1
  Bus Selector : BusSelector  OutputSignals=LP_CAN_RX.Shutdown_Data.High_AIR_Fault,LP_CAN_RX.Shutdown_Data.TSMS_Fault,LP_CAN_RX.Shutdown_Data.HVD_Fault,LP_CAN_RX.Shutdown_Data.Front_Return_Fault,LP_CAN_RX.Shutdown_Data.E2_Switch_Fault,LP_CAN_RX.Shutdown_Data.E1_Switch_Fault,LP_CAN_RX.Shutdown_Data.Latch_Out_Fault,LP_CAN_RX.Shutdown_Data.Latch_In_Fault,LP_CAN_RX.Shutdown_Data.BSPD_TSI_Fault,LP_CAN_RX.Shutdown_Data.BSPD_Fault,LP_CAN_RX.Shutdown_Data.IMD_Fault,LP_CAN_RX.Shutdown_Data.BMS_Fault,LP_CAN_RX.Shutdown_Data.ESTP_Right_Fault,LP_CAN_RX.Shutdown_Data.ESTP_Left_Fault
  Logical Operator : Logic  Operator=OR  Inputs=14  AllPortsSameDT=off  OutDataTypeStr=boolean
  Out1 : Outport
  wires:
  In1/1 -> Bus Selector/1
  Bus Creator/1 -> Out1/1
  Logical Operator/1 -> Bus Creator/1  "Shutdown_Error"
  Bus Selector/14 -> Logical Operator/14  "<ESTP_Left_Fault>"
  Bus Selector/13 -> Logical Operator/13  "<ESTP_Right_Fault>"
  Bus Selector/12 -> Logical Operator/12  "<BMS_Fault>"
  Bus Selector/11 -> Logical Operator/11  "<IMD_Fault>"
  Bus Selector/10 -> Logical Operator/10  "<BSPD_Fault>"
  Bus Selector/9 -> Logical Operator/9  "<BSPD_TSI_Fault>"
  Bus Selector/8 -> Logical Operator/8  "<Latch_In_Fault>"
  Bus Selector/7 -> Logical Operator/7  "<Latch_Out_Fault>"
  Bus Selector/6 -> Logical Operator/6  "<E1_Switch_Fault>"
  Bus Selector/5 -> Logical Operator/5  "<E2_Switch_Fault>"
  Bus Selector/4 -> Logical Operator/4  "<Front_Return_Fault>"
  Bus Selector/3 -> Logical Operator/3  "<HVD_Fault>"
  Bus Selector/2 -> Logical Operator/2  "<TSMS_Fault>"
  Bus Selector/1 -> Logical Operator/1  "<High_AIR_Fault>"

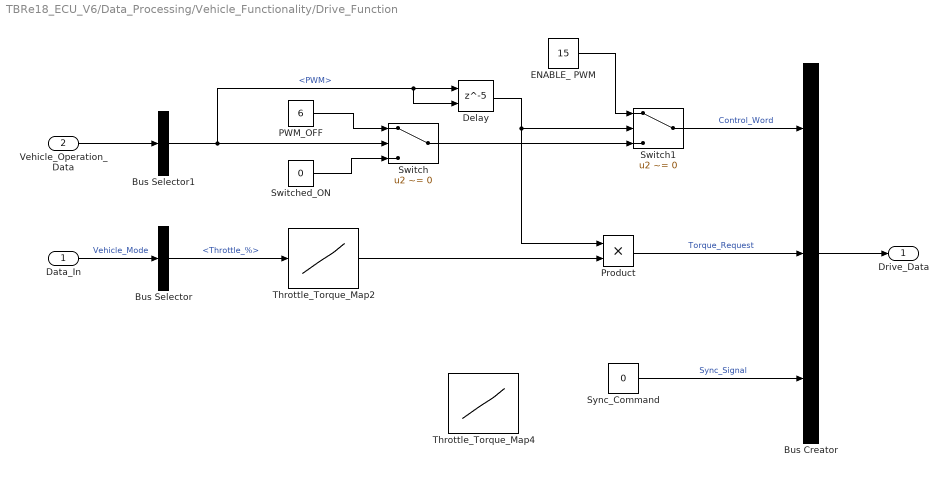
== system TBRe18_ECU_V6/Data_Processing/Vehicle_Functionality/Drive_Function ==
  Data_In : Inport
  Vehicle_Operation_Data : Inport  Port=2
  Bus Creator : BusCreator  Inputs=3
  Bus Selector : BusSelector  OutputSignals=ECU_IO_Data.Pedal_Box_Data.Throttle_%
  Bus Selector1 : BusSelector  OutputSignals=PWM
  Delay : Delay  DelayLength=5  ExternalReset=Falling
      settings: InputPortMap=u0,r5
  ENABLE_ PWM : Constant  Value=15  OutDataTypeStr=uint16
  PWM_OFF : Constant  Value=6  OutDataTypeStr=uint16
  Product : Product  OutDataTypeStr=int16
  Switch : Switch  Criteria=u2 ~= 0  OutDataTypeStr=uint16
  Switch1 : Switch  Criteria=u2 ~= 0  OutDataTypeStr=uint16
  Switched_ON : Constant  Value=0  OutDataTypeStr=uint16
  "Sync_Command " : Constant  Value=0  OutDataTypeStr=uint8  SampleTime=-1
  Throttle_Torque_Map2 : Lookup_n-D  NumberOfTableDimensions=1  BreakpointsForDimension1=[0,30,75,100]  Table=[0,30,400,500]  ExtrapMethod=Clip  UseLastTableValue=on  InternalRulePriority=Speed  OutDataTypeStr=uint16  RndMeth=Simplest  InputSameDT=on
  Throttle_Torque_Map4 : Lookup_n-D  NumberOfTableDimensions=1  BreakpointsForDimension1=[0,30,75,100]  Table=[0,100,600,750]  ExtrapMethod=Clip  UseLastTableValue=on  InternalRulePriority=Speed  OutDataTypeStr=uint16  RndMeth=Simplest  InputSameDT=on
  Drive_Data : Outport
  wires:
  "Sync_Command "/1 -> Bus Creator/3  "Sync_Signal"
  PWM_OFF/1 -> Switch/1
  Switched_ON/1 -> Switch/3
  Switch/1 -> Switch1/3
  ENABLE_ PWM/1 -> Switch1/1
  Delay/1 -> Product/1, Switch1/2
  Switch1/1 -> Bus Creator/1  "Control_Word"
  Bus Creator/1 -> Drive_Data/1
  Product/1 -> Bus Creator/2  "Torque_Request"
  Data_In/1 -> Bus Selector/1  "Vehicle_Mode"
  Vehicle_Operation_Data/1 -> Bus Selector1/1
  Bus Selector1/1 -> Delay/2, Delay/1, Switch/2  "<PWM>"
  Bus Selector/1 -> Throttle_Torque_Map2/1  "<Throttle_%>"
  Throttle_Torque_Map2/1 -> Product/2

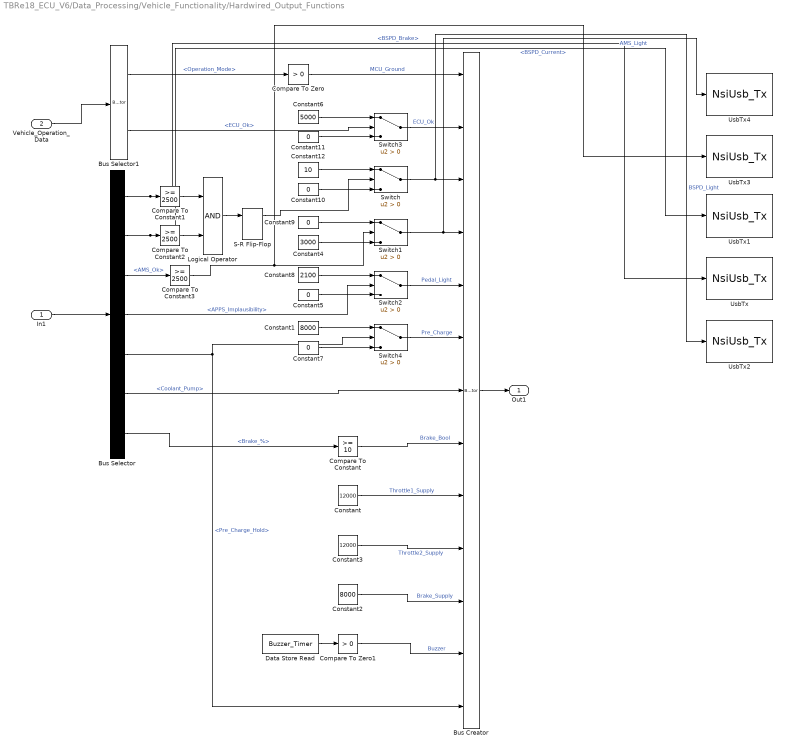
== system TBRe18_ECU_V6/Data_Processing/Vehicle_Functionality/Hardwired_Output_Functions ==
  In1 : Inport
  Vehicle_Operation_Data : Inport  Port=2
  Bus Creator : BusCreator  Inputs=13
  Bus Selector : BusSelector  OutputSignals=Raw_Input_Data.Hardwired_Inputs.Pedal_Box_Data.BSPD_Brake,Raw_Input_Data.Hardwired_Inputs.Pedal_Box_Data.BSPD_Current,Raw_Input_Data.Hardwired_Inputs.AMS_Ok,ECU_IO_Data.Pedal_Box_Data.APPS_Implausibility,BMS_Data.Pre_Charge_Hold,MCU_Data.Coolant_Pump,ECU_IO_Data.Pedal_Box_Data.Brake_%
  Bus Selector1 : BusSelector  OutputSignals=Operation_Mode,ECU_Ok
  Compare To Constant : simulink/Logic and Bit Operations/Compare To Constant  relop=>=  const=10  OutDataTypeStr=boolean
  Compare To Constant1 : simulink/Logic and Bit Operations/Compare To Constant  relop=>=  const=2500  OutDataTypeStr=boolean
  Compare To Constant2 : simulink/Logic and Bit Operations/Compare To Constant  relop=>=  const=2500  OutDataTypeStr=boolean
  Compare To Constant3 : simulink/Logic and Bit Operations/Compare To Constant  relop=>=  const=2500  OutDataTypeStr=boolean
  Compare To Zero : simulink/Logic and Bit Operations/Compare To Zero  relop=>  OutDataTypeStr=boolean
  Compare To Zero1 : simulink/Logic and Bit Operations/Compare To Zero  relop=>  OutDataTypeStr=boolean
  Constant : Constant  Value=12000  OutDataTypeStr=uint16
  Constant1 : Constant  Value=8000  OutDataTypeStr=Inherit: Inherit via back propagation
  Constant{5,9..11} (4 alike) : Constant  Value=0  OutDataTypeStr=uint16
  Constant12 : Constant  Value=10  OutDataTypeStr=uint16
  Constant2 : Constant  Value=8000  OutDataTypeStr=uint16
  Constant3 : Constant  Value=12000  OutDataTypeStr=uint16
  Constant4 : Constant  Value=3000  OutDataTypeStr=uint16
  Constant6 : Constant  Value=5000  OutDataTypeStr=uint16
  Constant7 : Constant  Value=0  OutDataTypeStr=Inherit: Inherit via back propagation
  Constant8 : Constant  Value=2100  OutDataTypeStr=uint16
  Data Store Read : DataStoreRead  DataStoreName=Buzzer_Timer
  Logical Operator : Logic  AllPortsSameDT=off  OutDataTypeStr=boolean
  S-R Flip-Flop : simulink_extras/Flip Flops/S-R Flip-Flop  initial_condition=0
  Switch : Switch  Criteria=u2 > Threshold  OutDataTypeStr=uint8
  Switch1 : Switch  Criteria=u2 > Threshold  OutDataTypeStr=uint8
  Switch2 : Switch  Criteria=u2 > Threshold
  Switch3 : Switch  Criteria=u2 > Threshold
  Switch4 : Switch  Criteria=u2 > Threshold  OutDataTypeStr=uint16
  UsbTx : S-Function  FunctionName=NsiUsb_Tx  Parameters=signame,resolution,offset,unite  SFunctionDeploymentMode=off  EnableBusSupport=off  mask(MUXlink Usb Tx){signame=BSPD_Brake, resolution=1, offset=0, unite=Bool}
      mask prompts: signame "Signal name ?"; resolution "Resolution ?"; offset "Offset ?"; unite "Unit ?"
      mask help: Transmit a frame on the USB Channel.
      mask init:
      | NsiUsb_Tx_InitializationFcn();
      settings: OpenFcn=NsiUsb_Tx_OpenFcn();
      mask Help:
      | eval('block=get_param(gcb, ''RTWdata'');')
      | web([docroot '\toolbox\MUXlink\html\blocks/' block.MUXlink_BlockType '.html'])
      mask Callback signame: NsiUsb_Tx_ApplyFcn(1);
      mask Callback resolution: NsiUsb_Tx_ApplyFcn(2);
      mask Callback offset: NsiUsb_Tx_ApplyFcn(3);
      mask Callback unite: NsiUsb_Tx_ApplyFcn(4);
      mask Display: image(imread('nsi.bmp'));text(0.5, 0.2, 'USB Tx', 'horizontalAlignment', 'center', 'verticalAlignment', 'base');plot([0.05 0.05 0.05 0.05 0.05 0.05 0.05 0.05 0.05 0.05]);port_label('input',1, 'BSPD_Brake');
  UsbTx1 : S-Function  FunctionName=NsiUsb_Tx  Parameters=signame,resolution,offset,unite  SFunctionDeploymentMode=off  EnableBusSupport=off  mask(MUXlink Usb Tx){signame=BSPD_Current, resolution=1, offset=0, unite=Bool}
      mask prompts: signame "Signal name ?"; resolution "Resolution ?"; offset "Offset ?"; unite "Unit ?"
      mask help: Transmit a frame on the USB Channel.
      mask init:
      | NsiUsb_Tx_InitializationFcn();
      settings: OpenFcn=NsiUsb_Tx_OpenFcn();
      mask Help:
      | eval('block=get_param(gcb, ''RTWdata'');')
      | web([docroot '\toolbox\MUXlink\html\blocks/' block.MUXlink_BlockType '.html'])
      mask Callback signame: NsiUsb_Tx_ApplyFcn(1);
      mask Callback resolution: NsiUsb_Tx_ApplyFcn(2);
      mask Callback offset: NsiUsb_Tx_ApplyFcn(3);
      mask Callback unite: NsiUsb_Tx_ApplyFcn(4);
      mask Display: image(imread('nsi.bmp'));text(0.5, 0.2, 'USB Tx', 'horizontalAlignment', 'center', 'verticalAlignment', 'base');plot([0.05 0.05 0.05 0.05 0.05 0.05 0.05 0.05 0.05 0.05]);port_label('input',1, 'BSPD_Current');
  UsbTx2 : S-Function  FunctionName=NsiUsb_Tx  Parameters=signame,resolution,offset,unite  SFunctionDeploymentMode=off  EnableBusSupport=off  mask(MUXlink Usb Tx){signame=BSPD_PWM Level, resolution=1, offset=0, unite=%}
      mask prompts: signame "Signal name ?"; resolution "Resolution ?"; offset "Offset ?"; unite "Unit ?"
      mask help: Transmit a frame on the USB Channel.
      mask init:
      | NsiUsb_Tx_InitializationFcn();
      settings: OpenFcn=NsiUsb_Tx_OpenFcn();
      mask Help:
      | eval('block=get_param(gcb, ''RTWdata'');')
      | web([docroot '\toolbox\MUXlink\html\blocks/' block.MUXlink_BlockType '.html'])
      mask Callback signame: NsiUsb_Tx_ApplyFcn(1);
      mask Callback resolution: NsiUsb_Tx_ApplyFcn(2);
      mask Callback offset: NsiUsb_Tx_ApplyFcn(3);
      mask Callback unite: NsiUsb_Tx_ApplyFcn(4);
      mask Display: image(imread('nsi.bmp'));text(0.5, 0.2, 'USB Tx', 'horizontalAlignment', 'center', 'verticalAlignment', 'base');plot([0.05 0.05 0.05 0.05 0.05 0.05 0.05 0.05 0.05 0.05]);port_label('input',1, 'BSPD_PWM Level');
  UsbTx3 : S-Function  FunctionName=NsiUsb_Tx  Parameters=signame,resolution,offset,unite  SFunctionDeploymentMode=off  EnableBusSupport=off  mask(MUXlink Usb Tx){signame=AMS_Ok, resolution=1, offset=0, unite=Bool}
      mask prompts: signame "Signal name ?"; resolution "Resolution ?"; offset "Offset ?"; unite "Unit ?"
      mask help: Transmit a frame on the USB Channel.
      mask init:
      | NsiUsb_Tx_InitializationFcn();
      settings: OpenFcn=NsiUsb_Tx_OpenFcn();
      mask Help:
      | eval('block=get_param(gcb, ''RTWdata'');')
      | web([docroot '\toolbox\MUXlink\html\blocks/' block.MUXlink_BlockType '.html'])
      mask Callback signame: NsiUsb_Tx_ApplyFcn(1);
      mask Callback resolution: NsiUsb_Tx_ApplyFcn(2);
      mask Callback offset: NsiUsb_Tx_ApplyFcn(3);
      mask Callback unite: NsiUsb_Tx_ApplyFcn(4);
      mask Display: image(imread('nsi.bmp'));text(0.5, 0.2, 'USB Tx', 'horizontalAlignment', 'center', 'verticalAlignment', 'base');plot([0.05 0.05 0.05 0.05 0.05 0.05 0.05 0.05 0.05 0.05]);port_label('input',1, 'AMS_Ok');
  UsbTx4 : S-Function  FunctionName=NsiUsb_Tx  Parameters=signame,resolution,offset,unite  SFunctionDeploymentMode=off  EnableBusSupport=off  mask(MUXlink Usb Tx){signame=AMS_Light, resolution=1, offset=0, unite=mV}
      mask prompts: signame "Signal name ?"; resolution "Resolution ?"; offset "Offset ?"; unite "Unit ?"
      mask help: Transmit a frame on the USB Channel.
      mask init:
      | NsiUsb_Tx_InitializationFcn();
      settings: OpenFcn=NsiUsb_Tx_OpenFcn();
      mask Help:
      | eval('block=get_param(gcb, ''RTWdata'');')
      | web([docroot '\toolbox\MUXlink\html\blocks/' block.MUXlink_BlockType '.html'])
      mask Callback signame: NsiUsb_Tx_ApplyFcn(1);
      mask Callback resolution: NsiUsb_Tx_ApplyFcn(2);
      mask Callback offset: NsiUsb_Tx_ApplyFcn(3);
      mask Callback unite: NsiUsb_Tx_ApplyFcn(4);
      mask Display: image(imread('nsi.bmp'));text(0.5, 0.2, 'USB Tx', 'horizontalAlignment', 'center', 'verticalAlignment', 'base');plot([0.05 0.05 0.05 0.05 0.05 0.05 0.05 0.05 0.05 0.05]);port_label('input',1, 'AMS_Light');
  Out1 : Outport
  wires:
  Constant/1 -> Bus Creator/9  "Throttle1_Supply"
  Bus Creator/1 -> Out1/1
  Constant2/1 -> Bus Creator/11  "Brake_Supply"
  Constant3/1 -> Bus Creator/10  "Throttle2_Supply"
  In1/1 -> Bus Selector/1
  Bus Selector/6 -> Bus Creator/7  "<Coolant_Pump>"
  Bus Selector/7 -> Compare To Constant/1  "<Brake_%>"
  Compare To Zero/1 -> Bus Creator/1  "MCU_Ground"
  Data Store Read/1 -> Compare To Zero1/1
  Compare To Zero1/1 -> Bus Creator/12  "Buzzer"
  Compare To Constant/1 -> Bus Creator/8  "Brake_Bool"
  Switch/1 -> UsbTx2/1, Bus Creator/3  "BSPD_Light"
  Switch1/1 -> UsbTx4/1, Bus Creator/4  "AMS_Light"
  Bus Selector/3 -> Compare To Constant3/1  "<AMS_Ok>"
  Bus Selector/4 -> Switch2/2  "<APPS_Implausibility>"
  Switch2/1 -> Bus Creator/5  "Pedal_Light"
  Switch4/1 -> Bus Creator/6  "Pre_Charge"
  Switch3/1 -> Bus Creator/2  "ECU_Ok"
  Constant1/1 -> Switch4/1
  Bus Selector/5 -> Switch4/2, Bus Creator/13  "<Pre_Charge_Hold>"
  Constant6/1 -> Switch3/1
  Constant7/1 -> Switch4/3
  Vehicle_Operation_Data/1 -> Bus Selector1/1
  Bus Selector1/1 -> Compare To Zero/1  "<Operation_Mode>"
  Bus Selector1/2 -> Switch3/2  "<ECU_Ok>"
  Constant5/1 -> Switch2/3
  Constant8/1 -> Switch2/1
  Constant4/1 -> Switch1/3
  Constant9/1 -> Switch1/1
  Constant10/1 -> Switch/3
  Constant11/1 -> Switch3/3
  Constant12/1 -> Switch/1
  Bus Selector/2 -> UsbTx1/1, Compare To Constant2/1  "<BSPD_Current>"
  Bus Selector/1 -> UsbTx/1, Compare To Constant1/1  "<BSPD_Brake>"
  Compare To Constant1/1 -> Logical Operator/1
  Compare To Constant2/1 -> Logical Operator/2
  Logical Operator/1 -> S-R Flip-Flop/1
  S-R Flip-Flop/1 -> Switch/2
  Compare To Constant3/1 -> UsbTx3/1, Switch1/2

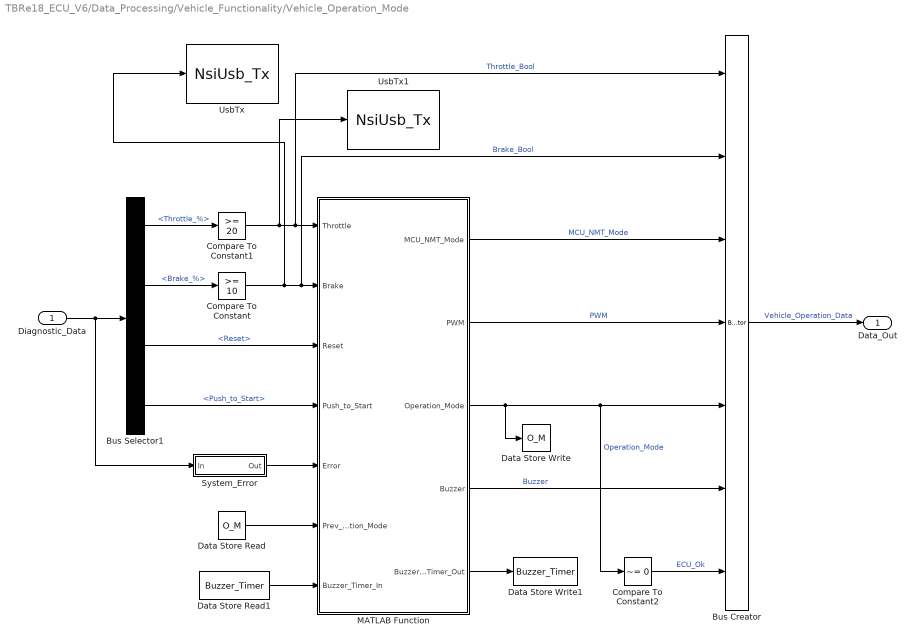
== system TBRe18_ECU_V6/Data_Processing/Vehicle_Functionality/Vehicle_Operation_Mode ==
  Diagnostic_Data : Inport
  Bus Creator : BusCreator  Inputs=7
  Bus Selector1 : BusSelector  OutputSignals=ECU_IO_Data.Pedal_Box_Data.Throttle_%,ECU_IO_Data.Pedal_Box_Data.Brake_%,Raw_Input_Data.Hardwired_Inputs.Console_Data.Reset,Raw_Input_Data.Hardwired_Inputs.Console_Data.Push_to_Start
  Compare To Constant : simulink/Logic and Bit Operations/Compare To Constant  relop=>=  const=10  OutDataTypeStr=boolean
  Compare To Constant1 : simulink/Logic and Bit Operations/Compare To Constant  relop=>=  const=20  OutDataTypeStr=boolean
  Compare To Constant2 : simulink/Logic and Bit Operations/Compare To Constant  relop=~=  const=0  OutDataTypeStr=boolean
  Data Store Read : DataStoreRead  DataStoreName=O_M
  Data Store Read1 : DataStoreRead  DataStoreName=Buzzer_Timer
  Data Store Write : DataStoreWrite  DataStoreName=O_M
  Data Store Write1 : DataStoreWrite  DataStoreName=Buzzer_Timer
  MATLAB Function : MATLAB Function  TreatAsAtomicUnit=on
  System_Error : Subsystem
  UsbTx : S-Function  FunctionName=NsiUsb_Tx  Parameters=signame,resolution,offset,unite  SFunctionDeploymentMode=off  EnableBusSupport=off  mask(MUXlink Usb Tx){signame=Brake_Bool, resolution=1, offset=0, unite=Bool}
      mask prompts: signame "Signal name ?"; resolution "Resolution ?"; offset "Offset ?"; unite "Unit ?"
      mask help: Transmit a frame on the USB Channel.
      mask init:
      | NsiUsb_Tx_InitializationFcn();
      settings: OpenFcn=NsiUsb_Tx_OpenFcn();
      mask Help:
      | eval('block=get_param(gcb, ''RTWdata'');')
      | web([docroot '\toolbox\MUXlink\html\blocks/' block.MUXlink_BlockType '.html'])
      mask Callback signame: NsiUsb_Tx_ApplyFcn(1);
      mask Callback resolution: NsiUsb_Tx_ApplyFcn(2);
      mask Callback offset: NsiUsb_Tx_ApplyFcn(3);
      mask Callback unite: NsiUsb_Tx_ApplyFcn(4);
      mask Display: image(imread('nsi.bmp'));text(0.5, 0.2, 'USB Tx', 'horizontalAlignment', 'center', 'verticalAlignment', 'base');plot([0.05 0.05 0.05 0.05 0.05 0.05 0.05 0.05 0.05 0.05]);port_label('input',1, 'Brake_Bool');
  UsbTx1 : S-Function  FunctionName=NsiUsb_Tx  Parameters=signame,resolution,offset,unite  SFunctionDeploymentMode=off  EnableBusSupport=off  mask(MUXlink Usb Tx){signame=Throttle_Bool, resolution=1, offset=0, unite=Bool}
      mask prompts: signame "Signal name ?"; resolution "Resolution ?"; offset "Offset ?"; unite "Unit ?"
      mask help: Transmit a frame on the USB Channel.
      mask init:
      | NsiUsb_Tx_InitializationFcn();
      settings: OpenFcn=NsiUsb_Tx_OpenFcn();
      mask Help:
      | eval('block=get_param(gcb, ''RTWdata'');')
      | web([docroot '\toolbox\MUXlink\html\blocks/' block.MUXlink_BlockType '.html'])
      mask Callback signame: NsiUsb_Tx_ApplyFcn(1);
      mask Callback resolution: NsiUsb_Tx_ApplyFcn(2);
      mask Callback offset: NsiUsb_Tx_ApplyFcn(3);
      mask Callback unite: NsiUsb_Tx_ApplyFcn(4);
      mask Display: image(imread('nsi.bmp'));text(0.5, 0.2, 'USB Tx', 'horizontalAlignment', 'center', 'verticalAlignment', 'base');plot([0.05 0.05 0.05 0.05 0.05 0.05 0.05 0.05 0.05 0.05]);port_label('input',1, 'Throttle_Bool');
  Data_Out : Outport
  wires:
  Bus Creator/1 -> Data_Out/1  "Vehicle_Operation_Data"
  Data Store Read/1 -> MATLAB Function/6(Prev_Operation_Mode)
  MATLAB Function/3(Operation_Mode) -> Data Store Write/1, Compare To Constant2/1, Bus Creator/5  "Operation_Mode"
  MATLAB Function/1(MCU_NMT_Mode) -> Bus Creator/3  "MCU_NMT_Mode"
  Diagnostic_Data/1 -> System_Error/1(In), Bus Selector1/1
  Bus Selector1/4 -> MATLAB Function/4(Push_to_Start)  "<Push_to_Start>"
  Bus Selector1/3 -> MATLAB Function/3(Reset)  "<Reset>"
  System_Error/1(Out) -> MATLAB Function/5(Error)
  MATLAB Function/2(PWM) -> Bus Creator/4  "PWM"
  Compare To Constant1/1 -> UsbTx1/1, Bus Creator/1, MATLAB Function/1(Throttle)  "Throttle_Bool"
  Compare To Constant/1 -> UsbTx/1, Bus Creator/2, MATLAB Function/2(Brake)  "Brake_Bool"
  Data Store Read1/1 -> MATLAB Function/7(Buzzer_Timer_In)
  MATLAB Function/5(Buzzer_Timer_Out) -> Data Store Write1/1
  MATLAB Function/4(Buzzer) -> Bus Creator/6  "Buzzer"
  Bus Selector1/1 -> Compare To Constant1/1  "<Throttle_%>"
  Bus Selector1/2 -> Compare To Constant/1  "<Brake_%>"
  Compare To Constant2/1 -> Bus Creator/7  "ECU_Ok"

== system TBRe18_ECU_V6/Data_Processing/Diagnostics/ECU_I//0s_Diagnostics/AIR ==
  note: AIR open = 0V
      | AIR closed = 5V
  note: Need additional info on the AIR
  In1 : Inport
  Bus Creator : BusCreator  Inputs=1
  Bus Selector : BusSelector  OutputSignals=AIR
  Compare To Zero : simulink/Logic and Bit Operations/Compare To Zero  relop===  OutDataTypeStr=boolean
  Out1 : Outport
  wires:
  Bus Creator/1 -> Out1/1
  In1/1 -> Bus Selector/1
  Bus Selector/1 -> Compare To Zero/1  "<AIR>"
  Compare To Zero/1 -> Bus Creator/1  "AIR_Error"

== system TBRe18_ECU_V6/Data_Processing/Diagnostics/ECU_I//0s_Diagnostics/IMD ==
  note: Need additional info on the IMD about level of frequency
      | Spec on x Drive:
  In1 : Inport
  Bus Creator : BusCreator  Inputs=1
  Bus Selector : BusSelector  OutputSignals=IMD_Frequency
  Compare To Zero : simulink/Logic and Bit Operations/Compare To Zero  relop===  OutDataTypeStr=boolean
  Out1 : Outport
  wires:
  Bus Creator/1 -> Out1/1
  In1/1 -> Bus Selector/1
  Bus Selector/1 -> Compare To Zero/1  "<IMD_Frequency>"
  Compare To Zero/1 -> Bus Creator/1  "ECU_IMD_Error"
